simulink model "q3_simulink"  (R2022a)
settings: Solver=VariableStepAuto  StartTime=0.0  StopTime=10  RelTol=1e-3
settings Model: Creator=Guilherme  LastModifiedBy=Guilherme

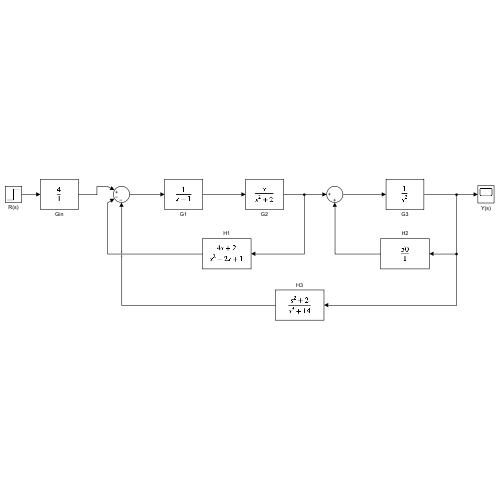
[thumbnail: Simulink's stored preview of the top-level diagram]
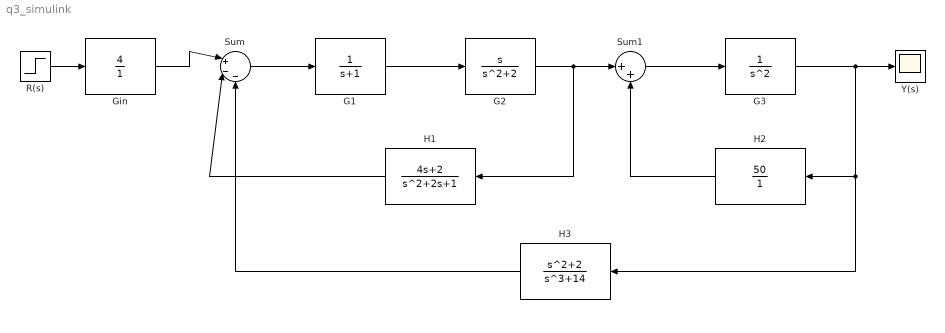
== system q3_simulink ==
  G1 : TransferFcn  Denominator=[1 1]
  G2 : TransferFcn  Numerator=[1 0]  Denominator=[1 0 2]
  G3 : TransferFcn  Denominator=[1 0 0]
  Gin : TransferFcn  Numerator=[4]  Denominator=[1]
  H1 : TransferFcn  Numerator=[4 2]
  H2 : TransferFcn  Numerator=[50]  Denominator=[1]
  H3 : TransferFcn  Numerator=[1 0 2]  Denominator=[1 0 0 14]
  R(s) : Step  SampleTime=0
  Sum : Sum  Inputs=|+--
  Sum1 : Sum  Inputs=|++
  Y(s) : Scope
  wires:
  Sum/1 -> G1/1
  H1/1 -> Sum/2
  R(s)/1 -> Gin/1
  Gin/1 -> Sum/1
  G2/1 -> H1/1, Sum1/1
  G1/1 -> G2/1
  Sum1/1 -> G3/1
  H2/1 -> Sum1/2
  G3/1 -> H3/1, H2/1, Y(s)/1
  H3/1 -> Sum/3
